simulink model "EV_Modeling"  (R2024b)
settings: Solver=FixedStepAuto  StartTime=0.0  StopTime=inf  FixedStep=0.1  RelTol=1e-3
values from neighbouring files (symbols this model uses):
  battery_SOC_resistance = battery_SOC(:,3)    [EV_Truck.m]
  battery_SOC_SOC = battery_SOC(:,1)    [EV_Truck.m]
  battery_SOC_voltage = battery_SOC(:,2)    [EV_Truck.m]
  motor_efficiency_efficiency = table2array(motor_efficiency(2:height(motor_efficiency),2:width(motor_efficiency)))    [EV_Truck.m]
  motor_efficiency_RPM = table2array(motor_efficiency(2:height(motor_efficiency),1))    [EV_Truck.m]
  motor_efficiency_torque = transpose(motor_efficiency_torque)    [EV_Truck.m]
  motor_RPM_torque = table2array(motor_torque(1:6,1))    [EV_Truck.m]
  motor_torque_RPM = table2array(motor_torque(1:6,2))    [EV_Truck.m]
undefined symbols (not defined in the file or in its folder): battery_builder_rtmsupport, DiscIntNeverNeededParam, gcbh, recurrentNet
libraries: simulink x8, fl_lib x6, nesl_utility x6, dlutilitylib x4, dlsequencelib x4, Batteries_lib x3, dlconvfclib x3, mpcadaslib x2, slpidlib x2, dlactivationlib x2, simulink_extras x1
(part 2 of 3)

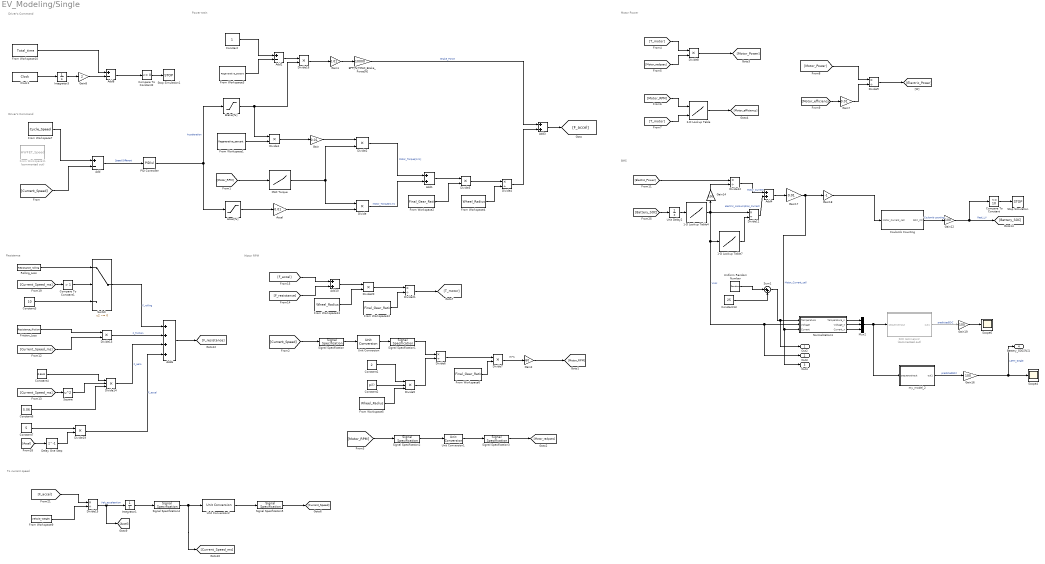
== system EV_Modeling/Single ==
  note: BMS
  note: To current speed
  note: Resistance
  note: Motor Power
  note: Power train
  note: Driver's Command
  note: RPS
  note: Motor RPM
  note: Driver's Command
  " Normalization1" : MATLAB Function  TreatAsAtomicUnit=on
  1-D Lookup Table4 : Lookup_n-D  NumberOfTableDimensions=1  BreakpointsForDimension1=battery_SOC_SOC  Table=battery_SOC_voltage  ExtrapMethod=Clip  UseLastTableValue=on  InternalRulePriority=Speed  RndMeth=Simplest
  1-D Lookup Table7 : Lookup_n-D  NumberOfTableDimensions=1  BreakpointsForDimension1=battery_SOC_SOC  Table=battery_SOC_resistance  InternalRulePriority=Speed  RndMeth=Simplest
  2-D Lookup Table : Lookup_n-D  BreakpointsForDimension1=motor_efficiency_RPM  BreakpointsForDimension2=motor_efficiency_torque  Table=motor_efficiency_efficiency  InternalRulePriority=Speed  RndMeth=Simplest
      settings: InputPortMap=u0,u1
  Accel : Gain  Gain=0.01
  Accel[%] : Saturate  UpperLimit=100  LowerLimit=0
  Add : Sum  Inputs=+-
  Add{1,3..4,10} (4 alike) : Sum
  Add2 : Sum  Inputs=+-
  Add6 : Sum  Inputs=++++
  Add8 : Sum  Inputs=+-
  BPP[%]*MAX_Brake_Force[N] : Gain  Gain=10000
  Brake[%] : Saturate  UpperLimit=0  LowerLimit=-100
  Clock1 : simulink_extras/Flip Flops/Clock  period=2
  Compare To Constant : simulink/Logic and Bit Operations/Compare To Constant  relop=<=  const=10  OutDataTypeStr=boolean
  Compare To Constant1 : simulink/Logic and Bit Operations/Compare To Constant  relop=>  const=1  OutDataTypeStr=boolean
  Compare To Constant2 : simulink/Logic and Bit Operations/Compare To Constant  relop=<=  const=0  OutDataTypeStr=boolean
  Constant : Constant
  Constant1 : Constant  Value=2
  Constant13 : Constant  Value=25
  Constant2 : Constant  Value=pi()
  Constant3 : Constant  Value=10
  Constant4 : Constant  Value=0.6441
  Constant6 : Constant  Value=5.06
  Constant7 : Constant  Value=5
  Coulomb Counting : Subsystem
  Delay One Step : Delay  DelayLength=1
  Divide{,1..3,7..8,13,16,19..20} (10 alike) : Product  Inputs=**
  Divide{4,6,9,11..12,15,21} (7 alike) : Product  Inputs=*/
  Divide14 : Product  Inputs=***
  Divide5 : Product  Inputs=***
  Friction_Loss : FromWorkspace  VariableName=Resistance_friction
  From Workspace1 : FromWorkspace  VariableName=Regenerative_percent
  From Workspace10 : FromWorkspace  VariableName=Total_time
  From Workspace11 : FromWorkspace  Commented=on  VariableName=HWFET_Speed
  From Workspace12 : FromWorkspace  VariableName=Final_Gear_Ratio
  From Workspace13 : FromWorkspace  VariableName=Wheel_Radius
  From Workspace2 : FromWorkspace  VariableName=Final_Gear_Ratio
  From Workspace3 : FromWorkspace  VariableName=Regenerative_percent
  From Workspace4 : FromWorkspace  VariableName=Wheel_Radius
  From Workspace5 : FromWorkspace  VariableName=Wheel_Radius
  From Workspace6 : FromWorkspace  VariableName=Final_Gear_Ratio
  From Workspace7 : FromWorkspace  VariableName=Cycle_Speed
  From Workspace9 : FromWorkspace  VariableName=Vehicle_Weight
  Gain{,1,7,17} (4 alike) : Gain  Gain=0.01
  Gain{12,14,16,19} (4 alike) : Gain  Gain=100
  Gain18 : Gain  Gain=-1
  Gain2 : Gain  Gain=60
  Gain8 : Gain  Gain=2
  Integrator1 : Integrator
  Integrator3 : Integrator
  MAX Torque : Lookup_n-D  NumberOfTableDimensions=1  BreakpointsForDimension1=motor_RPM_torque  Table=motor_torque_RPM  InternalRulePriority=Speed  RndMeth=Simplest
  Mux2 : Mux  Inputs=3
  PID Controller : slpidlib/PID Controller  Controller=PID  Form=Parallel  TimeDomain=Continuous-time  UseExternalTs=off  SampleTime=-1  IntegratorMethod=Forward Euler  FilterMethod=Forward Euler  ControllerParametersSource=internal  P=100  I=0.01  UseKiTs=off  D=0.0001  UseExternalDerivativeSource=off  N=10  UseFilter=on  TunerSelectOption=Transfer Function Based (PID Tuner App)  InitialConditionSource=internal  InitialConditionForIntegrator=0  InitialConditionForFilter=0  DifferentiatorICPrevScaledInput=0  ExternalReset=none  TrackingMode=off  Kt=1  LimitOutput=off  SatLimitsSource=internal  UpperSaturationLimit=inf  LowerSaturationLimit=-inf  LinearizeAsGain=on  AntiWindupMode=none  Kb=1  LimitIntegrator=off  UpperIntegratorSaturationLimit=inf  LowerIntegratorSaturationLimit=-inf  POutMin=[]  POutMax=[]  IOutMin=[]  IOutMax=[]  DOutMin=[]  DOutMax=[]  NOutMin=[]  NOutMax=[]  SumOutMin=[]  SumOutMax=[]  SaturationOutMin=[]  SaturationOutMax=[]  PParamMin=[]  PParamMax=[]  IParamMin=[]  IParamMax=[]  DParamMin=[]  DParamMax=[]  NParamMin=[]  NParamMax=[]  KbParamMin=[]  KbParamMax=[]  KtParamMin=[]  KtParamMax=[]  KbOutMin=[]  KbOutMax=[]  KtOutMin=[]  KtOutMax=[]  IntegratorOutMin=[]  IntegratorOutMax=[]  FilterOutMin=[]  FilterOutMax=[]  SumI1OutMin=[]  SumI1OutMax=[]  SumI2OutMin=[]  SumI2OutMax=[]  SumI3OutMin=[]  SumI3OutMax=[]  SumI4OutMin=[]  SumI4OutMax=[]  SumDOutMin=[]  SumDOutMax=[]  DifferentiatorOutMin=[]  DifferentiatorOutMax=[]  FilterDiffOutCoefMin=[]  FilterDiffOutCoefMax=[]  ReciprocalOutMin=[]  ReciprocalOutMax=[]  SumDenOutMin=[]  SumDenOutMax=[]  SumNumOutMin=[]  SumNumOutMax=[]  DivideOutMin=[]  DivideOutMax=[]  UdiffTsProdOutMin=[]  UdiffTsProdOutMax=[]  NTsProdOutMin=[]  NTsProdOutMax=[]  UintegralTsProdOutMin=[]  UintegralTsProdOutMax=[]  UngainTsProdOutMin=[]  UngainTsProdOutMax=[]  ClampingZeroOutDataTypeStr=Inherit: Inherit via back propagation  ClampingZeroOutMin=[]  ClampingZeroOutMax=[]  FilterDenConstantOutDataTypeStr=Inherit: Inherit via back propagation  FilterDenConstantOutMin=[]  FilterDenConstantOutMax=[]  PCopyOutDataTypeStr=Inherit: Inherit via back propagation  PCopyOutMin=[]  PCopyOutMax=[]  NCopyOutDataTypeStr=Inherit: Inherit via back propagation  NCopyOutMin=[]  NCopyOutMax=[]  IntegratorContinuousStateAttributes=''  IntegratorStateMustResolveToSignalObject=off  IntegratorRTWStateStorageClass=Auto  FilterContinuousStateAttributes=''  FilterStateMustResolveToSignalObject=off  FilterRTWStateStorageClass=Auto  ParallelPVariant=InternalParameters  IdealPVariant=Disabled  IVariant=InternalParameters  DVariant=InternalParameters  IntegratorVariant=Continuous  SatVariant=Disabled  AWVariant=Passthrough  PCopyVariant=Disabled  TRVariant=Disabled  FdbkBlocksVariant=Forward  IdealPFdbkVariant=Disabled  SatFdbkVariant=Disabled  DerivativeFilterVariant=ContFilter  NVariant=InternalParameters  NCopyVariant=Disabled  FilterICVariant=InternalICsFilter  IntegratorICVariant=InternalICs  ExternalResetVariant=Disabled  TRSumVariant=Passthrough  SumFdbkVariant=Disabled  SumVariant=Sum_PID  TsampFilterVariant=InternalTs  TsampNgainVariant=Passthrough  TsampIntegralVariant=Disabled_SignalSpec  ExternalSaturationOutDataTypeStr=Inherit: Same as second input  DerivativeSourceVariant=ErrorSignal  PreIntVariant=InternalPreInt
  Rolling_Loss : FromWorkspace  VariableName=Resistance_rolling
  SOC Estimator2 : Subsystem  Commented=on  TreatAsAtomicUnit=on
  Scope4 : Scope
  Scope6 : Scope
  Signal Specification : SignalSpecification  Unit=km/hr
  Signal Specification1 : SignalSpecification  Unit=m/s
  Signal Specification2 : SignalSpecification  Unit=rpm
  Signal Specification3 : SignalSpecification  Unit=rad/s
  Signal Specification4 : SignalSpecification  Unit=m/s
  Signal Specification5 : SignalSpecification  Unit=km/hr
  Square : Math  Operator=square
  Stop Simulation : Stop
  Stop Simulation1 : Stop
  Sum1 : Sum  Inputs=|++
  Switch : Switch  Criteria=u2 ~= 0  SaturateOnIntegerOverflow=off  InputSameDT=off
  Uniform Random Number : UniformRandomNumber  Minimum=0  Maximum=20  SampleTime=0.1
  Unit Conversion : UnitConversion
  Unit Conversion1 : UnitConversion
  Unit Conversion2 : UnitConversion
  Unit Delay2 : UnitDelay  SampleTime=-1  HasFrameUpgradeWarning=on
  my_model_2 : Subsystem
  Out2 : Outport
  Out3 : Outport  Port=2
  Out4 : Outport  Port=3
  Battery_SOC[%]1 : Outport  Port=4
  wires:
  Friction_Loss/1 -> Divide13/1
  Signal Specification3/1 -> [Motor_radpsec]
  From Workspace5/1 -> Divide5/3
  Divide1/1 -> Gain/1
  [Motor_RPM] -> Signal Specification2/1
  Divide/1 -> Add1/2  "Motor_Torque[N.m]"
  Divide7/1 -> Gain2/1
  Constant3/1 -> Switch/3
  Signal Specification5/1 -> [Current_Speed]
  Brake[%]/1 -> Divide16/2, Divide1/1
  Accel/1 -> Divide/2
  Compare To Constant1/1 -> Switch/2
  Switch/1 -> Add6/1  "F_rolling"
  [Current_Speed] -> Add/2
  MAX Torque/1 -> Divide2/2, Divide/1
  From Workspace1/1 -> Divide1/2
  Divide4/1 -> Add3/2
  Constant1/1 -> Divide5/1
  Rolling_Loss/1 -> Switch/1
  [T_motor] -> Divide8/1
  From Workspace9/1 -> Divide15/2
  Divide16/1 -> Gain1/1
  From Workspace3/1 -> Add2/2
  From Workspace4/1 -> Divide4/2
  Divide14/1 -> Add6/3  "F_aero"
  Add1/1 -> Divide3/1
  Add2/1 -> Divide16/1
  Divide8/1 -> [Motor_Power]
  From Workspace10/1 -> Add8/1
  [T_motor] -> 2-D Lookup Table/2
  Signal Specification/1 -> Unit Conversion/1
  Divide6/1 -> Divide7/1
  [F_accel] -> Divide15/1
  Divide3/1 -> Divide4/1
  Add/1 -> PID Controller/1  "Speed Different"
  [Motor_RPM] -> 2-D Lookup Table/1
  [Motor_Power] -> Divide9/1
  Accel[%]/1 -> Accel/1
  Gain7/1 -> Divide9/2
  Constant/1 -> Add2/1
  [Current_Speed_ms] -> Square/1
  Divide5/1 -> Divide6/2
  [Current_Speed] -> Signal Specification/1
  2-D Lookup Table/1 -> [Motor_efficiency]
  BPP[%]*MAX_Brake_Force[N]/1 -> Add3/1  "Brake_Force"
  Clock1/1 -> Integrator3/1
  [Current_Speed_ms] -> Compare To Constant1/1
  Divide9/1 -> [Electric_Power]
  Add3/1 -> [F_accel]
  Divide15/1 -> [Accel], Integrator1/1  "Veh_acceleartion"
  Add8/1 -> Compare To Constant2/1
  [Motor_RPM] -> MAX Torque/1
  Gain8/1 -> Add8/2
  Gain2/1 -> [Motor_RPM]
  Integrator3/1 -> Gain8/1
  Unit Conversion2/1 -> Signal Specification5/1
  Unit Conversion1/1 -> Signal Specification3/1
  Constant2/1 -> Divide5/2
  PID Controller/1 -> Brake[%]/1, Accel[%]/1  "Acceleration"
  Unit Conversion/1 -> Signal Specification1/1
  [Motor_efficiency] -> Gain7/1
  Signal Specification1/1 -> Divide6/1
  Divide2/1 -> Add1/1  "Motor_Torque[N.m]"
  Compare To Constant2/1 -> Stop Simulation1/1
  [Motor_radpsec] -> Divide8/2
  Divide13/1 -> Add6/2  "F_friction"
  Gain1/1 -> BPP[%]*MAX_Brake_Force[N]/1
  From Workspace2/1 -> Divide3/2
  [Current_Speed_ms] -> Divide13/2
  From Workspace6/1 -> Divide7/2
  Integrator1/1 -> Signal Specification4/1
  Signal Specification2/1 -> Unit Conversion1/1
  Square/1 -> Divide14/2
  Gain/1 -> Divide2/1
  Constant6/1 -> Divide14/3
  [Accel] -> Delay One Step/1
  Constant7/1 -> Divide19/1
  Delay One Step/1 -> Divide19/2
  Divide19/1 -> Add6/4  "F_accel"
  Signal Specification4/1 -> [Current_Speed_ms], Unit Conversion2/1
  Constant4/1 -> Divide14/1
  Add6/1 -> [F_resistance]
  [F_accel] -> Add10/1
  [F_resistance] -> Add10/2
  Divide21/1 -> [T_motor]
  Divide20/1 -> Divide21/1
  Add10/1 -> Divide20/1
  From Workspace13/1 -> Divide20/2
  From Workspace12/1 -> Divide21/2
  From Workspace7/1 -> Add/1
  Gain17/1 -> Out4/1, " Normalization1"/3(Current), Gain18/1  "Motor_Current_cell"
  Unit Delay2/1 -> 1-D Lookup Table4/1
  [Battery_SOC] -> Unit Delay2/1
  [Electric_Power] -> Divide12/1
  Gain18/1 -> Coulomb Counting/1(Motor_Current_cell)
  1-D Lookup Table7/1 -> Divide11/2
  Constant13/1 -> Sum1/2
  Gain12/1 -> Compare To Constant/1, [Battery_SOC]  "Real_LV"
  Gain19/1 -> Scope6/1
  Mux2/1 -> my_model_2/1(sequenceinput), SOC Estimator2/1(sequenceinput)
  Add4/1 -> Gain17/1
  Uniform Random Number/1 -> Sum1/1
  Gain14/1 -> Divide12/2
  my_model_2/1(out1) -> Gain16/1  "predictedSOC"
  " Normalization1"/3(Current_n) -> Mux2/3
  " Normalization1"/2(Voltage_n) -> Mux2/2
  Compare To Constant/1 -> Stop Simulation/1
  Divide12/1 -> Add4/1  "Motor_Current"
  SOC Estimator2/1(out1) -> Gain19/1  "predictedSOC"
  Coulomb Counting/1(SOC_CC) -> Gain12/1  "Coulomb counting"
  Sum1/1 -> Out2/1, " Normalization1"/1(Temperature)
  " Normalization1"/1(Temperature_n) -> Mux2/1
  1-D Lookup Table4/1 -> 1-D Lookup Table7/1, Out3/1, " Normalization1"/2(Voltage), Gain14/1, Divide11/1  "Vsoc"
  Divide11/1 -> Add4/2  "electric_consumption_Current"
  Gain16/1 -> Scope4/1, Battery_SOC[%]1/1  "LSTM_Single"

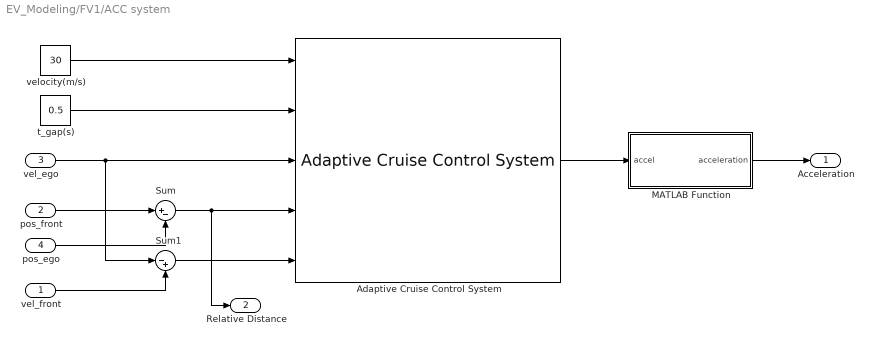
== system EV_Modeling/FV1/ACC system ==
  vel_front : Inport
  pos_front : Inport  Port=2
  vel_ego : Inport  Port=3
  pos_ego : Inport  Port=4
  Adaptive Cruise Control System : mpcadaslib/Adaptive Cruise Control System  EgoModel=tf(1,[0.5,1,0])  InitialEgoVelocity=20  DefaultSpacing=20  MaxVelocity=30  MinAcceleration=-3  amin_ext=off  MaxAcceleration=3  amax_ext=off  Ts=0.1  PredictionHorizon=100  ControllerBehavior=0.7  suboptimal=off  maxiter=10  datatypeopt=double  optmode=off  trackmode=off
      settings: LibrarySourceBlock=mpclib/Automated Driving/Adaptive Cruise Control System
  MATLAB Function : MATLAB Function  TreatAsAtomicUnit=on
  Sum : Sum  Inputs=|+-
  Sum1 : Sum  Inputs=|-+
  t_gap(s) : Constant  Value=0.5
  velocity(m/s) : Constant  Value=30
  Acceleration : Outport
  Relative Distance : Outport  Port=2
  wires:
  t_gap(s)/1 -> Adaptive Cruise Control System/2
  Sum/1 -> Relative Distance/1, Adaptive Cruise Control System/4
  Sum1/1 -> Adaptive Cruise Control System/5
  velocity(m/s)/1 -> Adaptive Cruise Control System/1
  Adaptive Cruise Control System/1 -> MATLAB Function/1(accel)
  pos_front/1 -> Sum/1
  pos_ego/1 -> Sum/2
  vel_front/1 -> Sum1/2
  vel_ego/1 -> Sum1/1, Adaptive Cruise Control System/3
  MATLAB Function/1(acceleration) -> Acceleration/1

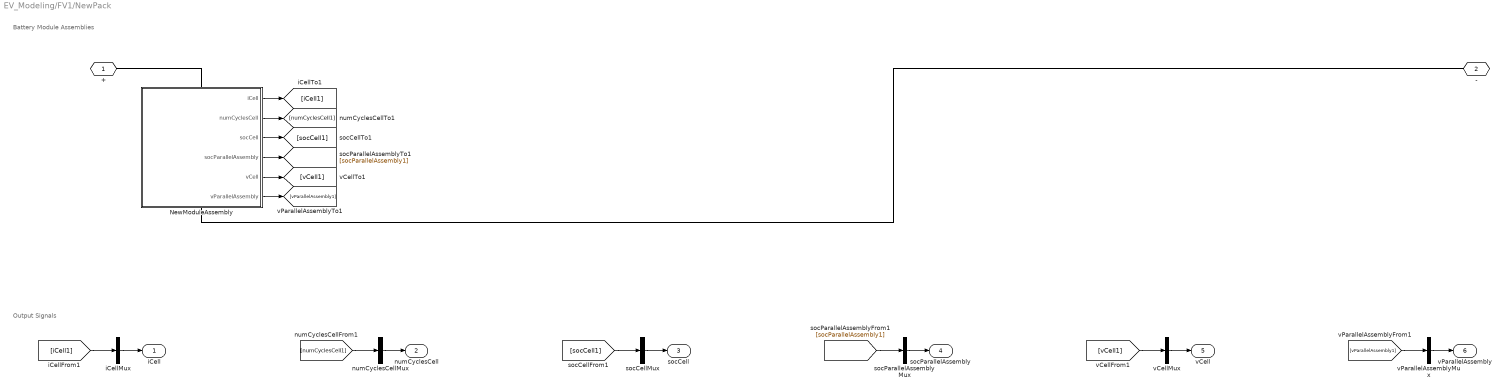
== system EV_Modeling/FV1/NewPack ==
  note: Battery Module Assemblies
  note: Output Signals
  NewModuleAssembly : Subsystem  LoadFcn=battery_builder_rtmsupport('loadfcn',gcbh);
      settings: CopyFcn=battery_builder_rtmsupport('copyfcn',gcbh);  PreCopyFcn=battery_builder_rtmsupport('precopyfcn',gcbh);  PreDeleteFcn=battery_builder_rtmsupport('predeletefcn',gcbh);  PortSchema="{\"entries\":[{\"content\":{\"sides\":[{\"content\":{\"connectorIds\":[\"LConn1\"]},\"type\":\"ConnectorPlacement.EquallySpacedRectSide\",\"uuid\":\"1202e0a0-be56-4819-949f-0e575ff0fad5\"},{\"content\":{\"connectorIds\":[\"RConn1\"],\"side\":\"RIGHT\"},\"type\":\"ConnectorPlacement.EquallySpacedRectSide\",\"uuid\":\"c846b010-7318-4529-a495-49262266c279\"},{\"content\":{\"side\":\"TOP\"},\"type\":\"ConnectorPlacement.EquallySpacedRectSide\",\"uuid\":\"5cadc0b8-a7f2-47b4-97e8-4fab1bc2ac7d\"},{\"content\":{\"connectorIds\":[\"Out1\",\"Out2\",\"Out3\",\"Out4\",\"Out5\",\"Out6\"],\"side\":\"BOTTOM\"},\"type\":\"ConnectorPlacement.EquallySpacedRectSide\",\"uuid\":\"9f2ef959-f133-4a8d-a7c5-293375a4069f\"}]},\"type\":\"ConnectorPlacement.EquallySpacedConnector\",\"uuid\":\"4d056c7c-5936-459e-9daf-456b1978dca2\"}],\"packageUris\":[\"http://schema.mathworks.com/mf0/Connector/R2020b\"],\"version\":\"1.0\"}"
      mask Display: image('$imagefile')
  iCellMux : Mux  Inputs=1
  numCyclesCellMux : Mux  Inputs=1
  socCellMux : Mux  Inputs=1
  socParallelAssemblyMux : Mux  Inputs=1
  vCellMux : Mux  Inputs=1
  vParallelAssemblyMux : Mux  Inputs=1
  + : PMIOPort  Side=Left
  - : PMIOPort  Port=2  Side=Right
  iCell : Outport
  numCyclesCell : Outport  Port=2
  socCell : Outport  Port=3
  socParallelAssembly : Outport  Port=4
  vCell : Outport  Port=5
  vParallelAssembly : Outport  Port=6
  wires:
  NewModuleAssembly/1(iCell) -> [iCell1]
  iCellMux/1 -> iCell/1
  [iCell1] -> iCellMux/1
  NewModuleAssembly/2(numCyclesCell) -> [numCyclesCell1]
  numCyclesCellMux/1 -> numCyclesCell/1
  [numCyclesCell1] -> numCyclesCellMux/1
  NewModuleAssembly/3(socCell) -> [socCell1]
  socCellMux/1 -> socCell/1
  [socCell1] -> socCellMux/1
  NewModuleAssembly/4(socParallelAssembly) -> [socParallelAssembly1]
  socParallelAssemblyMux/1 -> socParallelAssembly/1
  [socParallelAssembly1] -> socParallelAssemblyMux/1
  NewModuleAssembly/5(vCell) -> [vCell1]
  vCellMux/1 -> vCell/1
  [vCell1] -> vCellMux/1
  NewModuleAssembly/6(vParallelAssembly) -> [vParallelAssembly1]
  vParallelAssemblyMux/1 -> vParallelAssembly/1
  [vParallelAssembly1] -> vParallelAssemblyMux/1
  connections:
  NewModuleAssembly/LConn1 -- +/RConn1
  NewModuleAssembly/RConn1 -- -/RConn1

== system EV_Modeling/FV2/ACC system ==
  vel_front : Inport
  pos_front : Inport  Port=2
  vel_ego : Inport  Port=3
  pos_ego : Inport  Port=4
  Adaptive Cruise Control System : mpcadaslib/Adaptive Cruise Control System  EgoModel=tf(1,[0.5,1,0])  InitialEgoVelocity=20  DefaultSpacing=20  MaxVelocity=30  MinAcceleration=-3  amin_ext=off  MaxAcceleration=3  amax_ext=off  Ts=0.1  PredictionHorizon=100  ControllerBehavior=0.7  suboptimal=off  maxiter=10  datatypeopt=double  optmode=off  trackmode=off
  MATLAB Function : MATLAB Function  TreatAsAtomicUnit=on
  Sum : Sum  Inputs=|+-
  Sum1 : Sum  Inputs=|-+
  t_gap(s) : Constant  Value=0.5
  velocity(m/s) : Constant  Value=30
  Acceleration : Outport
  Relative Distance : Outport  Port=2
  wires:
  t_gap(s)/1 -> Adaptive Cruise Control System/2
  Sum/1 -> Relative Distance/1, Adaptive Cruise Control System/4
  Sum1/1 -> Adaptive Cruise Control System/5
  velocity(m/s)/1 -> Adaptive Cruise Control System/1
  Adaptive Cruise Control System/1 -> MATLAB Function/1(accel)
  pos_front/1 -> Sum/1
  pos_ego/1 -> Sum/2
  vel_front/1 -> Sum1/2
  vel_ego/1 -> Sum1/1, Adaptive Cruise Control System/3
  MATLAB Function/1(acceleration) -> Acceleration/1

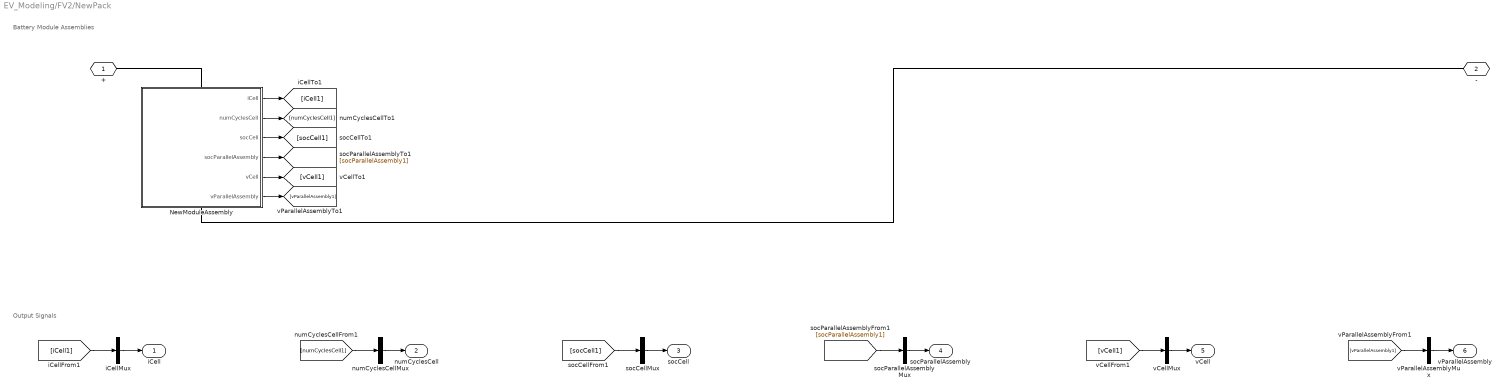
== system EV_Modeling/FV2/NewPack ==
  note: Battery Module Assemblies
  note: Output Signals
  NewModuleAssembly : Subsystem  LoadFcn=battery_builder_rtmsupport('loadfcn',gcbh);
      settings: CopyFcn=battery_builder_rtmsupport('copyfcn',gcbh);  PreCopyFcn=battery_builder_rtmsupport('precopyfcn',gcbh);  PreDeleteFcn=battery_builder_rtmsupport('predeletefcn',gcbh);  PortSchema="{\"entries\":[{\"content\":{\"sides\":[{\"content\":{\"connectorIds\":[\"LConn1\"]},\"type\":\"ConnectorPlacement.EquallySpacedRectSide\",\"uuid\":\"1202e0a0-be56-4819-949f-0e575ff0fad5\"},{\"content\":{\"connectorIds\":[\"RConn1\"],\"side\":\"RIGHT\"},\"type\":\"ConnectorPlacement.EquallySpacedRectSide\",\"uuid\":\"c846b010-7318-4529-a495-49262266c279\"},{\"content\":{\"side\":\"TOP\"},\"type\":\"ConnectorPlacement.EquallySpacedRectSide\",\"uuid\":\"5cadc0b8-a7f2-47b4-97e8-4fab1bc2ac7d\"},{\"content\":{\"connectorIds\":[\"Out1\",\"Out2\",\"Out3\",\"Out4\",\"Out5\",\"Out6\"],\"side\":\"BOTTOM\"},\"type\":\"ConnectorPlacement.EquallySpacedRectSide\",\"uuid\":\"9f2ef959-f133-4a8d-a7c5-293375a4069f\"}]},\"type\":\"ConnectorPlacement.EquallySpacedConnector\",\"uuid\":\"4d056c7c-5936-459e-9daf-456b1978dca2\"}],\"packageUris\":[\"http://schema.mathworks.com/mf0/Connector/R2020b\"],\"version\":\"1.0\"}"
      mask Display: image('$imagefile')
  iCellMux : Mux  Inputs=1
  numCyclesCellMux : Mux  Inputs=1
  socCellMux : Mux  Inputs=1
  socParallelAssemblyMux : Mux  Inputs=1
  vCellMux : Mux  Inputs=1
  vParallelAssemblyMux : Mux  Inputs=1
  + : PMIOPort  Side=Left
  - : PMIOPort  Port=2  Side=Right
  iCell : Outport
  numCyclesCell : Outport  Port=2
  socCell : Outport  Port=3
  socParallelAssembly : Outport  Port=4
  vCell : Outport  Port=5
  vParallelAssembly : Outport  Port=6
  wires:
  NewModuleAssembly/1(iCell) -> [iCell1]
  iCellMux/1 -> iCell/1
  [iCell1] -> iCellMux/1
  NewModuleAssembly/2(numCyclesCell) -> [numCyclesCell1]
  numCyclesCellMux/1 -> numCyclesCell/1
  [numCyclesCell1] -> numCyclesCellMux/1
  NewModuleAssembly/3(socCell) -> [socCell1]
  socCellMux/1 -> socCell/1
  [socCell1] -> socCellMux/1
  NewModuleAssembly/4(socParallelAssembly) -> [socParallelAssembly1]
  socParallelAssemblyMux/1 -> socParallelAssembly/1
  [socParallelAssembly1] -> socParallelAssemblyMux/1
  NewModuleAssembly/5(vCell) -> [vCell1]
  vCellMux/1 -> vCell/1
  [vCell1] -> vCellMux/1
  NewModuleAssembly/6(vParallelAssembly) -> [vParallelAssembly1]
  vParallelAssemblyMux/1 -> vParallelAssembly/1
  [vParallelAssembly1] -> vParallelAssemblyMux/1
  connections:
  NewModuleAssembly/LConn1 -- +/RConn1
  NewModuleAssembly/RConn1 -- -/RConn1

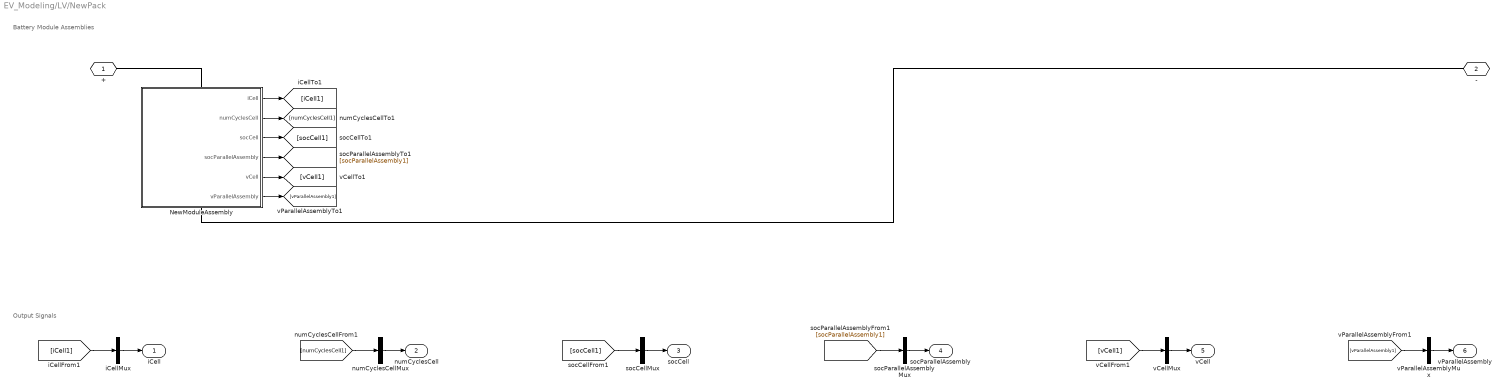
== system EV_Modeling/LV/NewPack ==
  note: Battery Module Assemblies
  note: Output Signals
  NewModuleAssembly : Subsystem  LoadFcn=battery_builder_rtmsupport('loadfcn',gcbh);
      settings: CopyFcn=battery_builder_rtmsupport('copyfcn',gcbh);  PreCopyFcn=battery_builder_rtmsupport('precopyfcn',gcbh);  PreDeleteFcn=battery_builder_rtmsupport('predeletefcn',gcbh);  PortSchema="{\"entries\":[{\"content\":{\"sides\":[{\"content\":{\"connectorIds\":[\"LConn1\"]},\"type\":\"ConnectorPlacement.EquallySpacedRectSide\",\"uuid\":\"1202e0a0-be56-4819-949f-0e575ff0fad5\"},{\"content\":{\"connectorIds\":[\"RConn1\"],\"side\":\"RIGHT\"},\"type\":\"ConnectorPlacement.EquallySpacedRectSide\",\"uuid\":\"c846b010-7318-4529-a495-49262266c279\"},{\"content\":{\"side\":\"TOP\"},\"type\":\"ConnectorPlacement.EquallySpacedRectSide\",\"uuid\":\"5cadc0b8-a7f2-47b4-97e8-4fab1bc2ac7d\"},{\"content\":{\"connectorIds\":[\"Out1\",\"Out2\",\"Out3\",\"Out4\",\"Out5\",\"Out6\"],\"side\":\"BOTTOM\"},\"type\":\"ConnectorPlacement.EquallySpacedRectSide\",\"uuid\":\"9f2ef959-f133-4a8d-a7c5-293375a4069f\"}]},\"type\":\"ConnectorPlacement.EquallySpacedConnector\",\"uuid\":\"4d056c7c-5936-459e-9daf-456b1978dca2\"}],\"packageUris\":[\"http://schema.mathworks.com/mf0/Connector/R2020b\"],\"version\":\"1.0\"}"
      mask Display: image('$imagefile')
  iCellMux : Mux  Inputs=1
  numCyclesCellMux : Mux  Inputs=1
  socCellMux : Mux  Inputs=1
  socParallelAssemblyMux : Mux  Inputs=1
  vCellMux : Mux  Inputs=1
  vParallelAssemblyMux : Mux  Inputs=1
  + : PMIOPort  Side=Left
  - : PMIOPort  Port=2  Side=Right
  iCell : Outport
  numCyclesCell : Outport  Port=2
  socCell : Outport  Port=3
  socParallelAssembly : Outport  Port=4
  vCell : Outport  Port=5
  vParallelAssembly : Outport  Port=6
  wires:
  NewModuleAssembly/1(iCell) -> [iCell1]
  iCellMux/1 -> iCell/1
  [iCell1] -> iCellMux/1
  NewModuleAssembly/2(numCyclesCell) -> [numCyclesCell1]
  numCyclesCellMux/1 -> numCyclesCell/1
  [numCyclesCell1] -> numCyclesCellMux/1
  NewModuleAssembly/3(socCell) -> [socCell1]
  socCellMux/1 -> socCell/1
  [socCell1] -> socCellMux/1
  NewModuleAssembly/4(socParallelAssembly) -> [socParallelAssembly1]
  socParallelAssemblyMux/1 -> socParallelAssembly/1
  [socParallelAssembly1] -> socParallelAssemblyMux/1
  NewModuleAssembly/5(vCell) -> [vCell1]
  vCellMux/1 -> vCell/1
  [vCell1] -> vCellMux/1
  NewModuleAssembly/6(vParallelAssembly) -> [vParallelAssembly1]
  vParallelAssemblyMux/1 -> vParallelAssembly/1
  [vParallelAssembly1] -> vParallelAssemblyMux/1
  connections:
  NewModuleAssembly/LConn1 -- +/RConn1
  NewModuleAssembly/RConn1 -- -/RConn1

== system EV_Modeling/Single/Coulomb Counting ==
  Motor_Current_cell : Inport
  Constant13 : Constant
  Constant14 : Constant  Value=50*3600
  Discrete-Time Integrator : DiscreteIntegrator  SampleTime=-1  ICPrevOutput=DiscIntNeverNeededParam  ICPrevScaledInput=DiscIntNeverNeededParam
  Divide10 : Product  Inputs=*/
  Minus1 : Sum  Inputs=+-
  SOC_CC : Outport
  wires:
  Minus1/1 -> SOC_CC/1
  Motor_Current_cell/1 -> Discrete-Time Integrator/1
  Constant13/1 -> Minus1/1
  Divide10/1 -> Minus1/2
  Discrete-Time Integrator/1 -> Divide10/1
  Constant14/1 -> Divide10/2

== system EV_Modeling/Single/SOC Estimator2 ==
  sequenceinput : Inport  PortDimensions="[3  1]"
  my_model_placeholder : Subsystem
  out1 : Outport
  wires:
  my_model_placeholder/1(out1) -> out1/1
  sequenceinput/1 -> my_model_placeholder/1(sequenceinput)

== system EV_Modeling/Single/my_model_2 ==
  sequenceinput : Inport  PortDimensions="[3  1]"
  dropout_1 : dlutilitylib/Dropout Layer  SampleTime=-1
  dropout_2 : dlutilitylib/Dropout Layer  SampleTime=-1
  fc : dlconvfclib/Fully Connected Layer  Layer=recurrentNet.Layers(6)  OutMin=[]  OutMax=[]  WeightsDataTypeStr=Inherit: Inherit via back propagation  WeightsMin=[]  WeightsMax=[]  BiasDataTypeStr=Inherit: Inherit via back propagation  BiasMin=[]  BiasMax=[]  MatrixMultiplyMin=[]  MatrixMultiplyMax=[]  SampleTime=-1
      settings: DataFormat=CT
  layer : dlactivationlib/Sigmoid Layer  ApproximationMethod=None  OutMin=[]  OutMax=[]  SampleTime=-1
  lstm_1 : dlsequencelib/LSTM Layer  Layer=recurrentNet.Layers(2)  Stateful=on  ApproximationMethod=None  InputWeightsDataTypeStr=Inherit: Inherit via back propagation  InputWeightsMin=[]  InputWeightsMax=[]  RecurrentWeightsDataTypeStr=Inherit: Inherit via back propagation  RecurrentWeightsMin=[]  RecurrentWeightsMax=[]  BiasDataTypeStr=Inherit: Inherit via back propagation  BiasMin=[]  BiasMax=[]  InitialCellStateDataTypeStr=Inherit: Inherit via back propagation  InitialCellStateMin=[]  InitialCellStateMax=[]  CellStateMin=[]  CellStateMax=[]  InitialHiddenStateDataTypeStr=Inherit: Inherit via back propagation  InitialHiddenStateMin=[]  InitialHiddenStateMax=[]  HiddenStateMin=[]  HiddenStateMax=[]  InputWeightsMatrixMultiplyOutMin=[]  InputWeightsMatrixMultiplyOutMax=[]  RecurrentWeightsMatrixMultiplyOutMin=[]  RecurrentWeightsMatrixMultiplyOutMax=[]  LinearGateAddOutMin=[]  LinearGateAddOutMax=[]  CellStateProductOutMin=[]  CellStateProductOutMax=[]  SampleTime=-1
      settings: DataFormat=CT
  lstm_2 : dlsequencelib/LSTM Layer  Layer=recurrentNet.Layers(4)  Stateful=on  ApproximationMethod=None  InputWeightsDataTypeStr=Inherit: Inherit via back propagation  InputWeightsMin=[]  InputWeightsMax=[]  RecurrentWeightsDataTypeStr=Inherit: Inherit via back propagation  RecurrentWeightsMin=[]  RecurrentWeightsMax=[]  BiasDataTypeStr=Inherit: Inherit via back propagation  BiasMin=[]  BiasMax=[]  InitialCellStateDataTypeStr=Inherit: Inherit via back propagation  InitialCellStateMin=[]  InitialCellStateMax=[]  CellStateMin=[]  CellStateMax=[]  InitialHiddenStateDataTypeStr=Inherit: Inherit via back propagation  InitialHiddenStateMin=[]  InitialHiddenStateMax=[]  HiddenStateMin=[]  HiddenStateMax=[]  InputWeightsMatrixMultiplyOutMin=[]  InputWeightsMatrixMultiplyOutMax=[]  RecurrentWeightsMatrixMultiplyOutMin=[]  RecurrentWeightsMatrixMultiplyOutMax=[]  LinearGateAddOutMin=[]  LinearGateAddOutMax=[]  CellStateProductOutMin=[]  CellStateProductOutMax=[]  SampleTime=-1
      settings: DataFormat=CT
  out1 : Outport
  wires:
  fc/1 -> layer/1
  lstm_1/1 -> dropout_1/1
  dropout_1/1 -> lstm_2/1
  layer/1 -> out1/1
  sequenceinput/1 -> lstm_1/1
  dropout_2/1 -> fc/1
  lstm_2/1 -> dropout_2/1

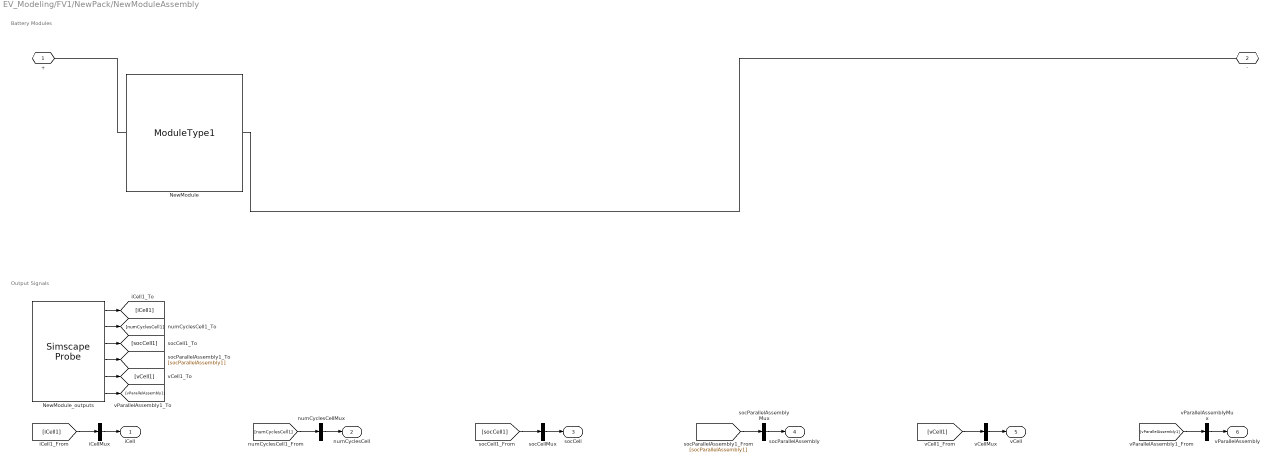
== system EV_Modeling/FV1/NewPack/NewModuleAssembly ==
  note: Output Signals
  note: Battery Modules
  NewModule : Batteries_lib/Modules/ModuleType1  SOC_vecCell=[0, .01, .02, .03, .04, .05, .06, .07, .08, .09, .1, .11, .12, .13, .14, .15, .16, .17, .18, .19, .2, .21, .22, .23, .24, .25, .26, .27, .28, .29, .3, .31, .32, .33, .34, .35, .36, .37, .38, .39, .4, .41, .42, .43, .44, .45, .46, .47, .48, .49, .5, .51, .52, .53, .54, .55, .56, .57, .58, .59, .6, .61, .62, .63, .64, .65, .66, .67, .68, .69, .7, .71, .72, .73, .74, .75, .76, .77, .78, .79, .8, .81, .82, .83, .84, .85, .86, .87, .88, .89, .9, .91, .92, .93, .94, .95, .96, .97, .98, .99, 1]  V0_vecCell=[35.84591, 36.10202, 36.35814, 36.61425, 36.87037, 37.12649, 37.3826, 37.63872, 37.89483, 38.09951, 38.20904, 38.28916, 38.37306, 38.42308, 38.45482, 38.47744, 38.49779, 38.54815, 38.5883, 38.63829, 38.68732, 38.72975, 38.77111, 38.80795, 38.83724, 38.8617, 38.89023, 38.9273, 38.96054, 38.98786, 39.01519, 39.03864, 39.06385, 39.08223, 39.1006, 39.11898, 39.13735, 39.15508, 39.16412, 39.17437, 39.18528, 39.19619, 39.20709, 39.21696, 39.22232, 39.22753, 39.23277, 39.23672, 39.23942, 39.24211, 39.24481, 39.24786, 39.25094, 39.2539, 39.25686, 39.26099, 39.26708, 39.27551, 39.28394, 39.29233, 39.30067, 39.31557, 39.33487, 39.35402, 39.37113, 39.38825, 39.40815, 39.43406, 39.46187, 39.48968, 39.51913, 39.55031, 39.5817, 39.60619, 39.62271, 39.63907, 39.65521, 39.67134, 39.68137, 39.69071, 39.70005, 39.7052, 39.70868, 39.70916, 39.70862, 39.70807, 39.70752, 39.71037, 39.72142, 39.72908, 39.73651, 39.73911, 39.73577, 39.72919, 39.73278, 39.7392, 39.74638, 39.75462, 39.8136, 40.01141, 40.30627] V  V_rangeCell=[27, Inf] V  R0_vecCell=[.47635, .41138, .35007, .29417, .24882, .2142, .18886, .17031, .1569, .14398, .13028, .11716, .10632, .09512, .08414, .07347, .06467, .05964, .05477, .05154, .04841, .04625, .04448, .04297, .04112, .03908, .0378, .03771, .03746, .03699, .03652, .03598, .03587, .03552, .03517, .03481, .03446, .03417, .03358, .03336, .03321, .03305, .0329, .0327, .03227, .03186, .03148, .03105, .03058, .03011, .02964, .02918, .02875, .02834, .02792, .02762, .02745, .02737, .02729, .02722, .02715, .0274, .02786, .0283, .02854, .02877, .02906, .02956, .03013, .0307, .03135, .03204, .03271, .03308, .03307, .03314, .03323, .03332, .03312, .03288, .03264, .03224, .03172, .03113, .03057, .03001, .02945, .02905, .02924, .0293, .02938, .02923, .02879, .02803, .02792, .02793, .02786, .02652, .02587, .02701, .00941] Ohm  AHCell=50.41 A*hr  extrapolation_optionCell=simscape.enum.extrapolation.nearest  P=18  S=18  iCell_specify=off  iCell_priority=None  iCell=0 A  iCell_nominal_specify=off  iCell_nominal_value=1  iCell_nominal_unit=A  vCell_specify=off  vCell_priority=None  vCell=0 V  vCell_nominal_specify=off  vCell_nominal_value=1  vCell_nominal_unit=V  socCell_specify=off  socCell_priority=High  socCell=1  socCell_nominal_specify=off  socCell_nominal_value=1  socCell_nominal_unit=1  numCyclesCell_specify=off  numCyclesCell_priority=High  numCyclesCell=0  numCyclesCell_nominal_specify=off  numCyclesCell_nominal_value=1  numCyclesCell_nominal_unit=1  vParallelAssembly_specify=off  vParallelAssembly_priority=None  vParallelAssembly=repmat(0, 18, 1) V  vParallelAssembly_nominal_specify=off  vParallelAssembly_nominal_value=1  vParallelAssembly_nominal_unit=V  socParallelAssembly_specify=off  socParallelAssembly_priority=None  socParallelAssembly=repmat(1, 18, 1)  socParallelAssembly_nominal_specify=off  socParallelAssembly_nominal_value=1  socParallelAssembly_nominal_unit=1
      settings: InternalSimscapePortConfiguration="{\"Bottom\":[{\"id\":\"n\",\"label\":\"-\",\"type\":\"foundation.electrical.electrical\"}],\"Left\":[],\"Right\":[],\"Top\":[{\"id\":\"p\",\"label\":\"+\",\"type\":\"foundation.electrical.electrical\"}]}"
  NewModule_outputs : SimscapeProbe  BoundBlock=7939  Variables="{\"iCell\":{\"Unit\":\"A\",\"PortLabel\":\"iCell\",\"Probing\":\"ON\"},\"numCyclesCell\":{\"Unit\":\"1\",\"PortLabel\":\"numCyclesCell\",\"Probing\":\"ON\"},\"socCell\":{\"Unit\":\"1\",\"PortLabel\":\"socCell\",\"Probing\":\"ON\"},\"socParallelAssembly\":{\"Unit\":\"1\",\"PortLabel\":\"socParallelAssembly\",\"Probing\":\"ON\"},\"vCell\":{\"Unit\":\"V\",\"PortLabel\":\"vCell\",\"Probing\":\"ON\"},\"vParallelAssembly\":{\"Unit\":\"V\",\"PortLabel\":\"vParallelAssembly\",\"Probing\":\"ON\"}}"
  iCellMux : Mux  Inputs=1
  numCyclesCellMux : Mux  Inputs=1
  socCellMux : Mux  Inputs=1
  socParallelAssemblyMux : Mux  Inputs=1
  vCellMux : Mux  Inputs=1
  vParallelAssemblyMux : Mux  Inputs=1
  + : PMIOPort  Side=Left
  - : PMIOPort  Port=2  Side=Right
  iCell : Outport
  numCyclesCell : Outport  Port=2
  socCell : Outport  Port=3
  socParallelAssembly : Outport  Port=4
  vCell : Outport  Port=5
  vParallelAssembly : Outport  Port=6
  wires:
  [vParallelAssembly1] -> vParallelAssemblyMux/1
  vParallelAssemblyMux/1 -> vParallelAssembly/1
  NewModule_outputs/6 -> [vParallelAssembly1]
  [vCell1] -> vCellMux/1
  vCellMux/1 -> vCell/1
  NewModule_outputs/5 -> [vCell1]
  [socParallelAssembly1] -> socParallelAssemblyMux/1
  socParallelAssemblyMux/1 -> socParallelAssembly/1
  NewModule_outputs/4 -> [socParallelAssembly1]
  [socCell1] -> socCellMux/1
  socCellMux/1 -> socCell/1
  NewModule_outputs/3 -> [socCell1]
  [numCyclesCell1] -> numCyclesCellMux/1
  numCyclesCellMux/1 -> numCyclesCell/1
  NewModule_outputs/2 -> [numCyclesCell1]
  [iCell1] -> iCellMux/1
  iCellMux/1 -> iCell/1
  NewModule_outputs/1 -> [iCell1]
  connections:
  NewModule/RConn1 -- -/RConn1
  NewModule/LConn1 -- +/RConn1

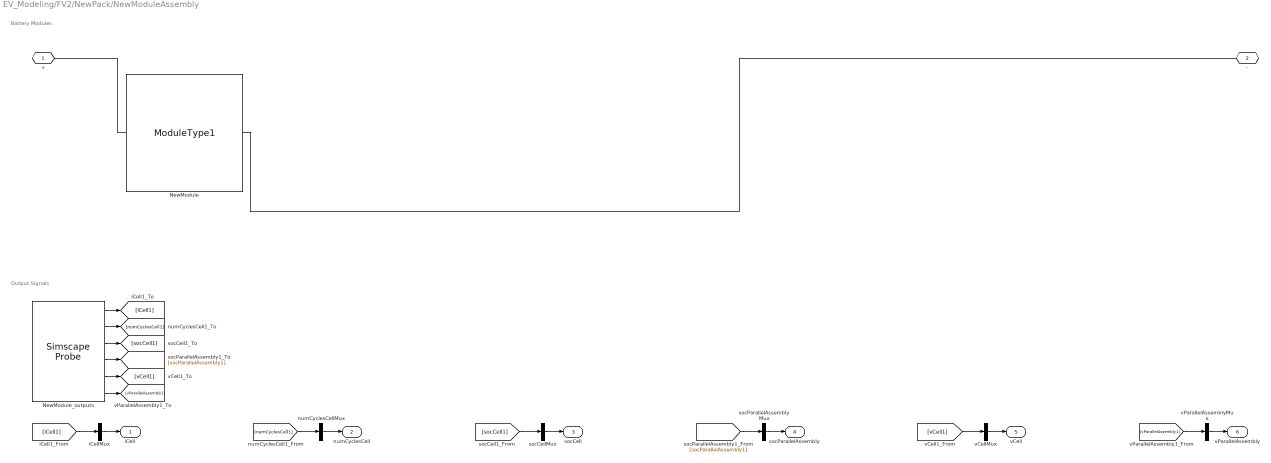
== system EV_Modeling/FV2/NewPack/NewModuleAssembly ==
  note: Output Signals
  note: Battery Modules
  NewModule : Batteries_lib/Modules/ModuleType1  SOC_vecCell=[0, .01, .02, .03, .04, .05, .06, .07, .08, .09, .1, .11, .12, .13, .14, .15, .16, .17, .18, .19, .2, .21, .22, .23, .24, .25, .26, .27, .28, .29, .3, .31, .32, .33, .34, .35, .36, .37, .38, .39, .4, .41, .42, .43, .44, .45, .46, .47, .48, .49, .5, .51, .52, .53, .54, .55, .56, .57, .58, .59, .6, .61, .62, .63, .64, .65, .66, .67, .68, .69, .7, .71, .72, .73, .74, .75, .76, .77, .78, .79, .8, .81, .82, .83, .84, .85, .86, .87, .88, .89, .9, .91, .92, .93, .94, .95, .96, .97, .98, .99, 1]  V0_vecCell=[35.84591, 36.10202, 36.35814, 36.61425, 36.87037, 37.12649, 37.3826, 37.63872, 37.89483, 38.09951, 38.20904, 38.28916, 38.37306, 38.42308, 38.45482, 38.47744, 38.49779, 38.54815, 38.5883, 38.63829, 38.68732, 38.72975, 38.77111, 38.80795, 38.83724, 38.8617, 38.89023, 38.9273, 38.96054, 38.98786, 39.01519, 39.03864, 39.06385, 39.08223, 39.1006, 39.11898, 39.13735, 39.15508, 39.16412, 39.17437, 39.18528, 39.19619, 39.20709, 39.21696, 39.22232, 39.22753, 39.23277, 39.23672, 39.23942, 39.24211, 39.24481, 39.24786, 39.25094, 39.2539, 39.25686, 39.26099, 39.26708, 39.27551, 39.28394, 39.29233, 39.30067, 39.31557, 39.33487, 39.35402, 39.37113, 39.38825, 39.40815, 39.43406, 39.46187, 39.48968, 39.51913, 39.55031, 39.5817, 39.60619, 39.62271, 39.63907, 39.65521, 39.67134, 39.68137, 39.69071, 39.70005, 39.7052, 39.70868, 39.70916, 39.70862, 39.70807, 39.70752, 39.71037, 39.72142, 39.72908, 39.73651, 39.73911, 39.73577, 39.72919, 39.73278, 39.7392, 39.74638, 39.75462, 39.8136, 40.01141, 40.30627] V  V_rangeCell=[27, Inf] V  R0_vecCell=[.47635, .41138, .35007, .29417, .24882, .2142, .18886, .17031, .1569, .14398, .13028, .11716, .10632, .09512, .08414, .07347, .06467, .05964, .05477, .05154, .04841, .04625, .04448, .04297, .04112, .03908, .0378, .03771, .03746, .03699, .03652, .03598, .03587, .03552, .03517, .03481, .03446, .03417, .03358, .03336, .03321, .03305, .0329, .0327, .03227, .03186, .03148, .03105, .03058, .03011, .02964, .02918, .02875, .02834, .02792, .02762, .02745, .02737, .02729, .02722, .02715, .0274, .02786, .0283, .02854, .02877, .02906, .02956, .03013, .0307, .03135, .03204, .03271, .03308, .03307, .03314, .03323, .03332, .03312, .03288, .03264, .03224, .03172, .03113, .03057, .03001, .02945, .02905, .02924, .0293, .02938, .02923, .02879, .02803, .02792, .02793, .02786, .02652, .02587, .02701, .00941] Ohm  AHCell=50.41 A*hr  extrapolation_optionCell=simscape.enum.extrapolation.nearest  P=18  S=18  iCell_specify=off  iCell_priority=None  iCell=0 A  iCell_nominal_specify=off  iCell_nominal_value=1  iCell_nominal_unit=A  vCell_specify=off  vCell_priority=None  vCell=0 V  vCell_nominal_specify=off  vCell_nominal_value=1  vCell_nominal_unit=V  socCell_specify=off  socCell_priority=High  socCell=1  socCell_nominal_specify=off  socCell_nominal_value=1  socCell_nominal_unit=1  numCyclesCell_specify=off  numCyclesCell_priority=High  numCyclesCell=0  numCyclesCell_nominal_specify=off  numCyclesCell_nominal_value=1  numCyclesCell_nominal_unit=1  vParallelAssembly_specify=off  vParallelAssembly_priority=None  vParallelAssembly=repmat(0, 18, 1) V  vParallelAssembly_nominal_specify=off  vParallelAssembly_nominal_value=1  vParallelAssembly_nominal_unit=V  socParallelAssembly_specify=off  socParallelAssembly_priority=None  socParallelAssembly=repmat(1, 18, 1)  socParallelAssembly_nominal_specify=off  socParallelAssembly_nominal_value=1  socParallelAssembly_nominal_unit=1
      settings: InternalSimscapePortConfiguration="{\"Bottom\":[{\"id\":\"n\",\"label\":\"-\",\"type\":\"foundation.electrical.electrical\"}],\"Left\":[],\"Right\":[],\"Top\":[{\"id\":\"p\",\"label\":\"+\",\"type\":\"foundation.electrical.electrical\"}]}"
  NewModule_outputs : SimscapeProbe  BoundBlock=8015  Variables="{\"iCell\":{\"Unit\":\"A\",\"PortLabel\":\"iCell\",\"Probing\":\"ON\"},\"numCyclesCell\":{\"Unit\":\"1\",\"PortLabel\":\"numCyclesCell\",\"Probing\":\"ON\"},\"socCell\":{\"Unit\":\"1\",\"PortLabel\":\"socCell\",\"Probing\":\"ON\"},\"socParallelAssembly\":{\"Unit\":\"1\",\"PortLabel\":\"socParallelAssembly\",\"Probing\":\"ON\"},\"vCell\":{\"Unit\":\"V\",\"PortLabel\":\"vCell\",\"Probing\":\"ON\"},\"vParallelAssembly\":{\"Unit\":\"V\",\"PortLabel\":\"vParallelAssembly\",\"Probing\":\"ON\"}}"
  iCellMux : Mux  Inputs=1
  numCyclesCellMux : Mux  Inputs=1
  socCellMux : Mux  Inputs=1
  socParallelAssemblyMux : Mux  Inputs=1
  vCellMux : Mux  Inputs=1
  vParallelAssemblyMux : Mux  Inputs=1
  + : PMIOPort  Side=Left
  - : PMIOPort  Port=2  Side=Right
  iCell : Outport
  numCyclesCell : Outport  Port=2
  socCell : Outport  Port=3
  socParallelAssembly : Outport  Port=4
  vCell : Outport  Port=5
  vParallelAssembly : Outport  Port=6
  wires:
  [vParallelAssembly1] -> vParallelAssemblyMux/1
  vParallelAssemblyMux/1 -> vParallelAssembly/1
  NewModule_outputs/6 -> [vParallelAssembly1]
  [vCell1] -> vCellMux/1
  vCellMux/1 -> vCell/1
  NewModule_outputs/5 -> [vCell1]
  [socParallelAssembly1] -> socParallelAssemblyMux/1
  socParallelAssemblyMux/1 -> socParallelAssembly/1
  NewModule_outputs/4 -> [socParallelAssembly1]
  [socCell1] -> socCellMux/1
  socCellMux/1 -> socCell/1
  NewModule_outputs/3 -> [socCell1]
  [numCyclesCell1] -> numCyclesCellMux/1
  numCyclesCellMux/1 -> numCyclesCell/1
  NewModule_outputs/2 -> [numCyclesCell1]
  [iCell1] -> iCellMux/1
  iCellMux/1 -> iCell/1
  NewModule_outputs/1 -> [iCell1]
  connections:
  NewModule/RConn1 -- -/RConn1
  NewModule/LConn1 -- +/RConn1

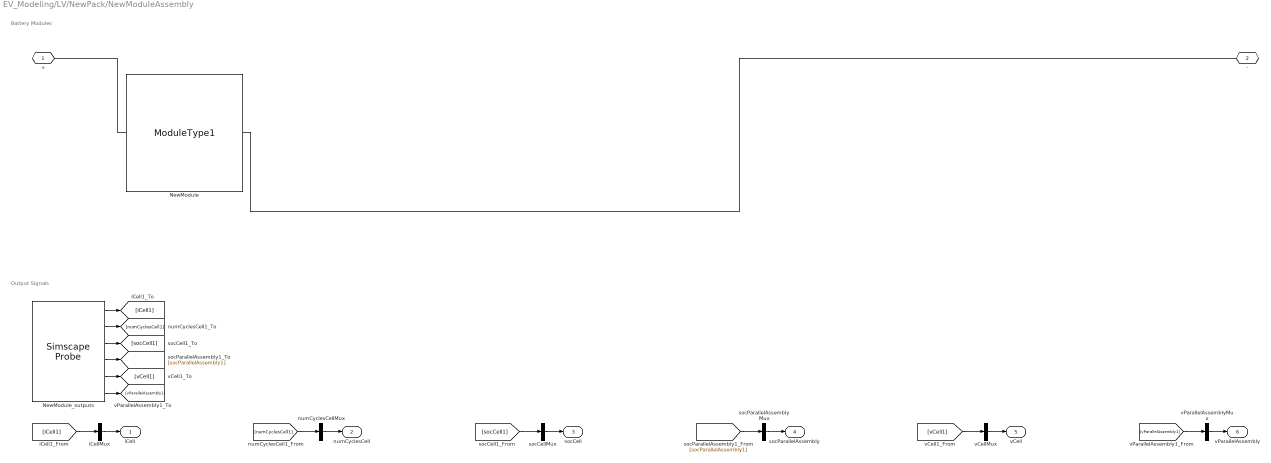
== system EV_Modeling/LV/NewPack/NewModuleAssembly ==
  note: Output Signals
  note: Battery Modules
  NewModule : Batteries_lib/Modules/ModuleType1  SOC_vecCell=[0, .01, .02, .03, .04, .05, .06, .07, .08, .09, .1, .11, .12, .13, .14, .15, .16, .17, .18, .19, .2, .21, .22, .23, .24, .25, .26, .27, .28, .29, .3, .31, .32, .33, .34, .35, .36, .37, .38, .39, .4, .41, .42, .43, .44, .45, .46, .47, .48, .49, .5, .51, .52, .53, .54, .55, .56, .57, .58, .59, .6, .61, .62, .63, .64, .65, .66, .67, .68, .69, .7, .71, .72, .73, .74, .75, .76, .77, .78, .79, .8, .81, .82, .83, .84, .85, .86, .87, .88, .89, .9, .91, .92, .93, .94, .95, .96, .97, .98, .99, 1]  V0_vecCell=[35.84591, 36.10202, 36.35814, 36.61425, 36.87037, 37.12649, 37.3826, 37.63872, 37.89483, 38.09951, 38.20904, 38.28916, 38.37306, 38.42308, 38.45482, 38.47744, 38.49779, 38.54815, 38.5883, 38.63829, 38.68732, 38.72975, 38.77111, 38.80795, 38.83724, 38.8617, 38.89023, 38.9273, 38.96054, 38.98786, 39.01519, 39.03864, 39.06385, 39.08223, 39.1006, 39.11898, 39.13735, 39.15508, 39.16412, 39.17437, 39.18528, 39.19619, 39.20709, 39.21696, 39.22232, 39.22753, 39.23277, 39.23672, 39.23942, 39.24211, 39.24481, 39.24786, 39.25094, 39.2539, 39.25686, 39.26099, 39.26708, 39.27551, 39.28394, 39.29233, 39.30067, 39.31557, 39.33487, 39.35402, 39.37113, 39.38825, 39.40815, 39.43406, 39.46187, 39.48968, 39.51913, 39.55031, 39.5817, 39.60619, 39.62271, 39.63907, 39.65521, 39.67134, 39.68137, 39.69071, 39.70005, 39.7052, 39.70868, 39.70916, 39.70862, 39.70807, 39.70752, 39.71037, 39.72142, 39.72908, 39.73651, 39.73911, 39.73577, 39.72919, 39.73278, 39.7392, 39.74638, 39.75462, 39.8136, 40.01141, 40.30627] V  V_rangeCell=[27, Inf] V  R0_vecCell=[.47635, .41138, .35007, .29417, .24882, .2142, .18886, .17031, .1569, .14398, .13028, .11716, .10632, .09512, .08414, .07347, .06467, .05964, .05477, .05154, .04841, .04625, .04448, .04297, .04112, .03908, .0378, .03771, .03746, .03699, .03652, .03598, .03587, .03552, .03517, .03481, .03446, .03417, .03358, .03336, .03321, .03305, .0329, .0327, .03227, .03186, .03148, .03105, .03058, .03011, .02964, .02918, .02875, .02834, .02792, .02762, .02745, .02737, .02729, .02722, .02715, .0274, .02786, .0283, .02854, .02877, .02906, .02956, .03013, .0307, .03135, .03204, .03271, .03308, .03307, .03314, .03323, .03332, .03312, .03288, .03264, .03224, .03172, .03113, .03057, .03001, .02945, .02905, .02924, .0293, .02938, .02923, .02879, .02803, .02792, .02793, .02786, .02652, .02587, .02701, .00941] Ohm  AHCell=50.41 A*hr  extrapolation_optionCell=simscape.enum.extrapolation.nearest  P=18  S=18  iCell_specify=off  iCell_priority=None  iCell=0 A  iCell_nominal_specify=off  iCell_nominal_value=1  iCell_nominal_unit=A  vCell_specify=off  vCell_priority=None  vCell=0 V  vCell_nominal_specify=off  vCell_nominal_value=1  vCell_nominal_unit=V  socCell_specify=off  socCell_priority=High  socCell=1  socCell_nominal_specify=off  socCell_nominal_value=1  socCell_nominal_unit=1  numCyclesCell_specify=off  numCyclesCell_priority=High  numCyclesCell=0  numCyclesCell_nominal_specify=off  numCyclesCell_nominal_value=1  numCyclesCell_nominal_unit=1  vParallelAssembly_specify=off  vParallelAssembly_priority=None  vParallelAssembly=repmat(0, 18, 1) V  vParallelAssembly_nominal_specify=off  vParallelAssembly_nominal_value=1  vParallelAssembly_nominal_unit=V  socParallelAssembly_specify=off  socParallelAssembly_priority=None  socParallelAssembly=repmat(1, 18, 1)  socParallelAssembly_nominal_specify=off  socParallelAssembly_nominal_value=1  socParallelAssembly_nominal_unit=1
      settings: InternalSimscapePortConfiguration="{\"Bottom\":[{\"id\":\"n\",\"label\":\"-\",\"type\":\"foundation.electrical.electrical\"}],\"Left\":[],\"Right\":[],\"Top\":[{\"id\":\"p\",\"label\":\"+\",\"type\":\"foundation.electrical.electrical\"}]}"
  NewModule_outputs : SimscapeProbe  BoundBlock=7866  Variables="{\"iCell\":{\"Unit\":\"A\",\"PortLabel\":\"iCell\",\"Probing\":\"ON\"},\"numCyclesCell\":{\"Unit\":\"1\",\"PortLabel\":\"numCyclesCell\",\"Probing\":\"ON\"},\"socCell\":{\"Unit\":\"1\",\"PortLabel\":\"socCell\",\"Probing\":\"ON\"},\"socParallelAssembly\":{\"Unit\":\"1\",\"PortLabel\":\"socParallelAssembly\",\"Probing\":\"ON\"},\"vCell\":{\"Unit\":\"V\",\"PortLabel\":\"vCell\",\"Probing\":\"ON\"},\"vParallelAssembly\":{\"Unit\":\"V\",\"PortLabel\":\"vParallelAssembly\",\"Probing\":\"ON\"}}"
  iCellMux : Mux  Inputs=1
  numCyclesCellMux : Mux  Inputs=1
  socCellMux : Mux  Inputs=1
  socParallelAssemblyMux : Mux  Inputs=1
  vCellMux : Mux  Inputs=1
  vParallelAssemblyMux : Mux  Inputs=1
  + : PMIOPort  Side=Left
  - : PMIOPort  Port=2  Side=Right
  iCell : Outport
  numCyclesCell : Outport  Port=2
  socCell : Outport  Port=3
  socParallelAssembly : Outport  Port=4
  vCell : Outport  Port=5
  vParallelAssembly : Outport  Port=6
  wires:
  [vParallelAssembly1] -> vParallelAssemblyMux/1
  vParallelAssemblyMux/1 -> vParallelAssembly/1
  NewModule_outputs/6 -> [vParallelAssembly1]
  [vCell1] -> vCellMux/1
  vCellMux/1 -> vCell/1
  NewModule_outputs/5 -> [vCell1]
  [socParallelAssembly1] -> socParallelAssemblyMux/1
  socParallelAssemblyMux/1 -> socParallelAssembly/1
  NewModule_outputs/4 -> [socParallelAssembly1]
  [socCell1] -> socCellMux/1
  socCellMux/1 -> socCell/1
  NewModule_outputs/3 -> [socCell1]
  [numCyclesCell1] -> numCyclesCellMux/1
  numCyclesCellMux/1 -> numCyclesCell/1
  NewModule_outputs/2 -> [numCyclesCell1]
  [iCell1] -> iCellMux/1
  iCellMux/1 -> iCell/1
  NewModule_outputs/1 -> [iCell1]
  connections:
  NewModule/RConn1 -- -/RConn1
  NewModule/LConn1 -- +/RConn1

== system EV_Modeling/Single/SOC Estimator2/my_model_placeholder ==
  sequenceinput : Inport  PortDimensions="[3  1]"
  dropout_1 : dlutilitylib/Dropout Layer  SampleTime=-1
  dropout_2 : dlutilitylib/Dropout Layer  SampleTime=-1
  fc_proj_in : dlconvfclib/Fully Connected Layer  Layer=recurrentNet.Layers(6)  OutMin=[]  OutMax=[]  WeightsDataTypeStr=Inherit: Inherit via back propagation  WeightsMin=[]  WeightsMax=[]  BiasDataTypeStr=Inherit: Inherit via back propagation  BiasMin=[]  BiasMax=[]  MatrixMultiplyMin=[]  MatrixMultiplyMax=[]  SampleTime=-1
      settings: DataFormat=CT
  fc_proj_out : dlconvfclib/Fully Connected Layer  Layer=recurrentNet.Layers(7)  OutMin=[]  OutMax=[]  WeightsDataTypeStr=Inherit: Inherit via back propagation  WeightsMin=[]  WeightsMax=[]  BiasDataTypeStr=Inherit: Inherit via back propagation  BiasMin=[]  BiasMax=[]  MatrixMultiplyMin=[]  MatrixMultiplyMax=[]  SampleTime=-1
      settings: DataFormat=CT
  layer : dlactivationlib/Sigmoid Layer  ApproximationMethod=None  OutMin=[]  OutMax=[]  OutDataTypeStr=Inherit: Inherit via back propagation  SampleTime=-1
  lstm_1 : dlsequencelib/LSTM Projected Layer  Layer=recurrentNet.Layers(2)  Stateful=on  ApproximationMethod=None  InputWeightsDataTypeStr=Inherit: Inherit via back propagation  InputWeightsMin=[]  InputWeightsMax=[]  RecurrentWeightsDataTypeStr=Inherit: Inherit via back propagation  RecurrentWeightsMin=[]  RecurrentWeightsMax=[]  BiasDataTypeStr=Inherit: Inherit via back propagation  BiasMin=[]  BiasMax=[]  InputProjectorWeightsDataTypeStr=Inherit: Inherit via back propagation  InputProjectorWeightsMin=[]  InputProjectorWeightsMax=[]  OutputProjectorWeightsDataTypeStr=Inherit: Inherit via back propagation  OutputProjectorWeightsMin=[]  OutputProjectorWeightsMax=[]  InitialCellStateDataTypeStr=Inherit: Inherit via back propagation  InitialCellStateMin=[]  InitialCellStateMax=[]  CellStateMin=[]  CellStateMax=[]  InitialHiddenStateDataTypeStr=Inherit: Inherit via back propagation  InitialHiddenStateMin=[]  InitialHiddenStateMax=[]  HiddenStateMin=[]  HiddenStateMax=[]  InputWeightsMatrixMultiplyOutMin=[]  InputWeightsMatrixMultiplyOutMax=[]  RecurrentWeightsMatrixMultiplyOutMin=[]  RecurrentWeightsMatrixMultiplyOutMax=[]  InputProjectorWeightsMatrixMultiplyOutMin=[]  InputProjectorWeightsMatrixMultiplyOutMax=[]  OutputProjectorWeightsMatrixMultiplyOutMin=[]  OutputProjectorWeightsMatrixMultiplyOutMax=[]  LinearGateAddOutMin=[]  LinearGateAddOutMax=[]  CellStateProductOutMin=[]  CellStateProductOutMax=[]  SampleTime=-1
      settings: DataFormat=CT
  lstm_2 : dlsequencelib/LSTM Projected Layer  Layer=recurrentNet.Layers(4)  Stateful=on  ApproximationMethod=None  InputWeightsDataTypeStr=Inherit: Inherit via back propagation  InputWeightsMin=[]  InputWeightsMax=[]  RecurrentWeightsDataTypeStr=Inherit: Inherit via back propagation  RecurrentWeightsMin=[]  RecurrentWeightsMax=[]  BiasDataTypeStr=Inherit: Inherit via back propagation  BiasMin=[]  BiasMax=[]  InputProjectorWeightsDataTypeStr=Inherit: Inherit via back propagation  InputProjectorWeightsMin=[]  InputProjectorWeightsMax=[]  OutputProjectorWeightsDataTypeStr=Inherit: Inherit via back propagation  OutputProjectorWeightsMin=[]  OutputProjectorWeightsMax=[]  InitialCellStateDataTypeStr=Inherit: Inherit via back propagation  InitialCellStateMin=[]  InitialCellStateMax=[]  CellStateMin=[]  CellStateMax=[]  InitialHiddenStateDataTypeStr=Inherit: Inherit via back propagation  InitialHiddenStateMin=[]  InitialHiddenStateMax=[]  HiddenStateMin=[]  HiddenStateMax=[]  InputWeightsMatrixMultiplyOutMin=[]  InputWeightsMatrixMultiplyOutMax=[]  RecurrentWeightsMatrixMultiplyOutMin=[]  RecurrentWeightsMatrixMultiplyOutMax=[]  InputProjectorWeightsMatrixMultiplyOutMin=[]  InputProjectorWeightsMatrixMultiplyOutMax=[]  OutputProjectorWeightsMatrixMultiplyOutMin=[]  OutputProjectorWeightsMatrixMultiplyOutMax=[]  LinearGateAddOutMin=[]  LinearGateAddOutMax=[]  CellStateProductOutMin=[]  CellStateProductOutMax=[]  SampleTime=-1
      settings: DataFormat=CT
  out1 : Outport
  wires:
  fc_proj_in/1 -> fc_proj_out/1
  lstm_2/1 -> dropout_2/1
  dropout_2/1 -> fc_proj_in/1
  fc_proj_out/1 -> layer/1
  sequenceinput/1 -> lstm_1/1
  layer/1 -> out1/1
  lstm_1/1 -> dropout_1/1
  dropout_1/1 -> lstm_2/1

== matlab function EV_Modeling/LV/Drag coefficient1 ==
  data: IVD input; C_drag output
function C_drag = fcn(IVD)
a = -0.1012;
b = -0.1002;
c = 0.6441;

C_drag = a * exp(b * (IVD-8)) + c;

== matlab function EV_Modeling/FV2/ACC system/MATLAB Function ==
  data: accel input; acceleration output
function acceleration  = fcn(accel)

if accel > 0 
    acceleration = (accel * 100)/0.15;
elseif accel < 0 
    acceleration = (accel * 100)/0.33;
else
    acceleration = 0; % accel이 0이거나 NaN일 경우에도 대응
end

== matlab function EV_Modeling/FV2/Drag coefficient ==
  data: IVD input; C_drag output
function C_drag = fcn(IVD)
a = -0.4629;
b = -0.068;
c = 0.6441;

C_drag = a * exp(b * (IVD-8)) + c;

== matlab function EV_Modeling/Single/ Normalization1 ==
  data: Temperature input; Temperature_n output; Voltage input; Voltage_n output; Current input; Current_n output
function [Temperature_n, Voltage_n, Current_n] = Normalization (Temperature, Voltage, Current)

minT = 25;
maxT = 45;
if (Temperature < minT) 
    Temperature = minT;
end
if (Temperature > maxT)
    Temperature = maxT;
end
Temperature_n = rescale(Temperature,InputMin=minT,InputMax=maxT);

minV = 3.1724;
maxV = 4.1679;
if (Voltage < minV) 
    Voltage = minV;
end
if (Voltage > maxV)
    Voltage = maxV;
end
Voltage_n = rescale(Voltage,InputMin=minV,InputMax=maxV);

minI = -1;
maxI = 7;
if (Current < minI) 
    Current = minI;
end
if (Current > maxI)
    Current = maxI;
end
Current_n = rescale(Current,InputMin=minI,InputMax=maxI);
